simulink subsystem "RT_RelativeWindOnBlade"  (R2025a)
settings: Solver=VariableStepAuto  StartTime=0.0  StopTime=10.0  RelTol=1e-3
undefined symbols (not defined in the file): RT_BEDistFromEffSta_A, RT_BladeSegment_P, RT_HubOffsetBody_P, RT_ShaftTiltFwd_P, RT_ShaftTiltRight_P
settings Model: DataDictionary=Rotor.sldd  EnableAccessToBaseWorkspace=off  DefaultTestHarness=RT_RelativeWindOnBlade_Harness  Creator=tunglt60  LastModifiedBy=tunglt60

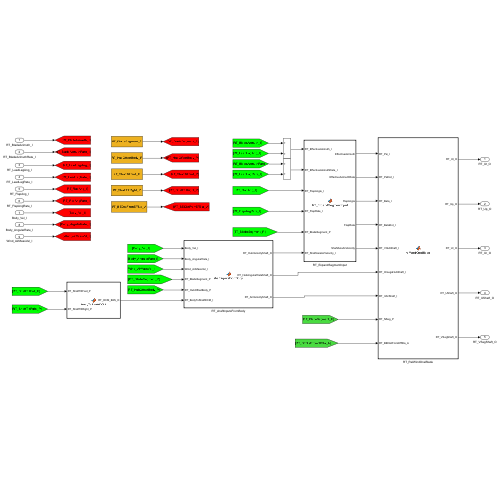
[thumbnail: Simulink's stored preview of the top-level diagram]
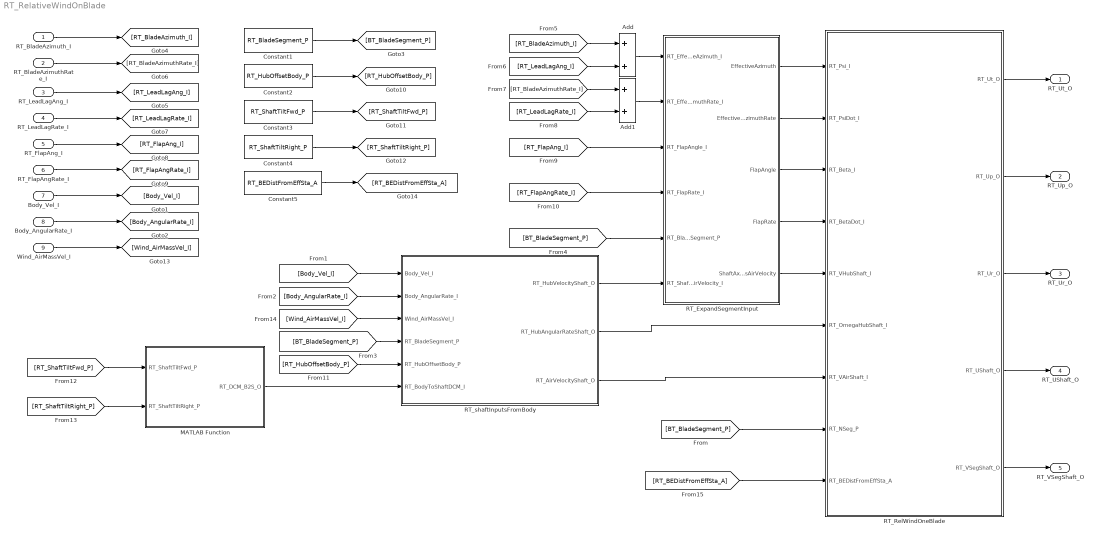
== system RT_RelativeWindOnBlade ==
  RT_BladeAzimuth_I : Inport
  RT_BladeAzimuthRate_I : Inport  Port=2
  RT_LeadLagAng_I : Inport  Port=3
  RT_LeadLagRate_I : Inport  Port=4
  RT_FlapAng_I : Inport  Port=5
  RT_FlapAngRate_I : Inport  Port=6
  Body_Vel_I : Inport  Port=7
  Body_AngularRate_I : Inport  Port=8
  Wind_AirMassVel_I : Inport  Port=9
  Add : Sum
  Add1 : Sum
  Constant1 : Constant  Value=RT_BladeSegment_P
  Constant2 : Constant  Value=RT_HubOffsetBody_P
  Constant3 : Constant  Value=RT_ShaftTiltFwd_P
  Constant4 : Constant  Value=RT_ShaftTiltRight_P
  Constant5 : Constant  Value=RT_BEDistFromEffSta_A
  MATLAB Function : MATLAB Function  TreatAsAtomicUnit=on
  RT_ExpandSegmentInput : MATLAB Function  TreatAsAtomicUnit=on
  RT_RelWindOneBlade : MATLAB Function  TreatAsAtomicUnit=on
  RT_shaftInputsFromBody : MATLAB Function  TreatAsAtomicUnit=on
  RT_Ut_O : Outport
  RT_Up_O : Outport  Port=2
  RT_Ur_O : Outport  Port=3
  RT_UShaft_O : Outport  Port=4
  RT_VSegShaft_O : Outport  Port=5
  wires:
  Add/1 -> RT_ExpandSegmentInput/1(RT_EffectiveAzimuth_I)
  Add1/1 -> RT_ExpandSegmentInput/2(RT_EffectiveAzimuthRate_I)
  Constant1/1 -> [BT_BladeSegment_P]
  [BT_BladeSegment_P] -> RT_ExpandSegmentInput/5(RT_BladeSegment_P)
  RT_BladeAzimuth_I/1 -> [RT_BladeAzimuth_I]
  RT_LeadLagRate_I/1 -> [RT_LeadLagRate_I]
  RT_FlapAngRate_I/1 -> [RT_FlapAngRate_I]
  RT_BladeAzimuthRate_I/1 -> [RT_BladeAzimuthRate_I]
  RT_LeadLagAng_I/1 -> [RT_LeadLagAng_I]
  RT_FlapAng_I/1 -> [RT_FlapAng_I]
  [RT_LeadLagAng_I] -> Add/2
  [RT_BladeAzimuth_I] -> Add/1
  [RT_BladeAzimuthRate_I] -> Add1/1
  [RT_LeadLagRate_I] -> Add1/2
  [RT_FlapAng_I] -> RT_ExpandSegmentInput/3(RT_FlapAngle_I)
  [RT_FlapAngRate_I] -> RT_ExpandSegmentInput/4(RT_FlapRate_I)
  Constant2/1 -> [RT_HubOffsetBody_P]
  Constant3/1 -> [RT_ShaftTiltFwd_P]
  Constant4/1 -> [RT_ShaftTiltRight_P]
  RT_ExpandSegmentInput/1(EffectiveAzimuth) -> RT_RelWindOneBlade/1(RT_Psi_I)
  RT_ExpandSegmentInput/2(EffectiveAzimuthRate) -> RT_RelWindOneBlade/2(RT_PsiDot_I)
  RT_ExpandSegmentInput/3(FlapAngle) -> RT_RelWindOneBlade/3(RT_Beta_I)
  RT_ExpandSegmentInput/4(FlapRate) -> RT_RelWindOneBlade/4(RT_BetaDot_I)
  [RT_ShaftTiltRight_P] -> MATLAB Function/2(RT_ShaftTiltRight_P)
  MATLAB Function/1(RT_DCM_B2S_O) -> RT_shaftInputsFromBody/6(RT_BodyToShaftDCM_I)
  [RT_ShaftTiltFwd_P] -> MATLAB Function/1(RT_ShaftTiltFwd_P)
  [BT_BladeSegment_P] -> RT_shaftInputsFromBody/4(RT_BladeSegment_P)
  [RT_HubOffsetBody_P] -> RT_shaftInputsFromBody/5(RT_HubOffsetBody_P)
  RT_shaftInputsFromBody/1(RT_HubVelocityShaft_O) -> RT_ExpandSegmentInput/6(RT_ShaftAxisAirVelocity_I)
  RT_shaftInputsFromBody/2(RT_HubAngularRateShaft_O) -> RT_RelWindOneBlade/6(RT_OmegaHubShaft_I)
  RT_shaftInputsFromBody/3(RT_AirVelocityShaft_O) -> RT_RelWindOneBlade/7(RT_VAirShaft_I)
  RT_ExpandSegmentInput/5(ShaftAxisAirVelocity) -> RT_RelWindOneBlade/5(RT_VHubShaft_I)
  [BT_BladeSegment_P] -> RT_RelWindOneBlade/8(RT_NSeg_P)
  Body_Vel_I/1 -> [Body_Vel_I]
  [Body_Vel_I] -> RT_shaftInputsFromBody/1(Body_Vel_I)
  Body_AngularRate_I/1 -> [Body_AngularRate_I]
  [Body_AngularRate_I] -> RT_shaftInputsFromBody/2(Body_AngularRate_I)
  [Wind_AirMassVel_I] -> RT_shaftInputsFromBody/3(Wind_AirMassVel_I)
  Wind_AirMassVel_I/1 -> [Wind_AirMassVel_I]
  [RT_BEDistFromEffSta_A] -> RT_RelWindOneBlade/9(RT_BEDistFromEffSta_A)
  Constant5/1 -> [RT_BEDistFromEffSta_A]
  RT_RelWindOneBlade/1(RT_Ut_O) -> RT_Ut_O/1
  RT_RelWindOneBlade/2(RT_Up_O) -> RT_Up_O/1
  RT_RelWindOneBlade/3(RT_Ur_O) -> RT_Ur_O/1
  RT_RelWindOneBlade/4(RT_UShaft_O) -> RT_UShaft_O/1
  RT_RelWindOneBlade/5(RT_VSegShaft_O) -> RT_VSegShaft_O/1

== matlab function RT_RelativeWindOnBlade/RT_shaftInputsFromBody ==
  data: Body_Vel_I input; RT_HubVelocityShaft_O output; Body_AngularRate_I input; Wind_AirMassVel_I input; RT_BladeSegment_P input; RT_HubAngularRateShaft_O output; RT_AirVelocityShaft_O output; RT_HubOffsetBody_P input; RT_BodyToShaftDCM_I input
function [RT_HubVelocityShaft_O, RT_HubAngularRateShaft_O, ...
    RT_AirVelocityShaft_O] = shaftInputsFromBody( ...
    Body_Vel_I, Body_AngularRate_I, ...
    Wind_AirMassVel_I, RT_BladeSegment_P, RT_HubOffsetBody_P, RT_BodyToShaftDCM_I)
%
% Convert body-axis quantities to shaft-axis quantities at rotor hub.
%
% Conventions:
%   body : x forward, y right, z down
%   shaft: z_s down along rotor shaft
%
% Inputs:
%   RT_ReferenceVelocityBody_I : [3x1], translational velocity of reference point
%                                in body axes (usually CG or body-origin)
%   RT_BodyAngularRate_I       : [3x1], body angular rate [p;q;r] in body axes
%   RT_AirMassVelocityBody_I   : [3x1] or [3xNSEG], air-mass velocity in body axes
%                                (NOT relative wind, NOT already minus vehicle velocity)
%   RT_BladeSegment_P
%   RT_HubOffsetBody_P      [3x1]
%   RT_BodyToShaftDCM_P     [3x3]
%
% Outputs:
%   RT_HubVelocityShaft_O      : [3x1], hub translational velocity in shaft axes
%   RT_HubAngularRateShaft_O   : [3x1], shaft angular rate in shaft axes
%   RT_AirVelocityShaft_O      : [3xNSEG], air-mass velocity in shaft axes
%
% Notes:
%   - If the reference point is already the hub, set:
%         RT_RotorParameter_I.RT_HubOffsetBody_P = [0;0;0]
%   - This assumes shaft is fixed to body.
%     If shaft rotates relative to body, add that relative rate separately.
%

NSEG = RT_BladeSegment_P;
C_SB   = RT_BodyToShaftDCM_I;
rHub_B = RT_HubOffsetBody_P;

% Hub translational velocity in body axes
Vhub_B = Body_Vel_I + cross(Body_AngularRate_I, rHub_B);

% Shaft fixed to body:
Whub_B = Body_AngularRate_I;

% Rotate to shaft axes
RT_HubVelocityShaft_O    = C_SB * Vhub_B;
RT_HubAngularRateShaft_O = C_SB * Whub_B;

% Air-mass velocity: expand to 3xNSEG if needed, then rotate each column
Vair_B = expand3xN(Wind_AirMassVel_I, NSEG);
RT_AirVelocityShaft_O = zeros(3, NSEG);

for k = 1:NSEG
    RT_AirVelocityShaft_O(:,k) = C_SB * Vair_B(:,k);
end

end

function Y = expand3xN(X, N)
%#codegen
if size(X,2) == 1
    Y = zeros(3, N);
    for i = 1:N
        Y(:,i) = X;
    end
else
    Y = X;
end
end

== matlab function RT_RelativeWindOnBlade/RT_RelWindOneBlade ==
  data: RT_Psi_I input; RT_Ut_O output; RT_PsiDot_I input; RT_Beta_I input; RT_BetaDot_I input; RT_VHubShaft_I input; RT_OmegaHubShaft_I input; RT_VAirShaft_I input; RT_NSeg_P input; RT_Up_O output; RT_Ur_O output; RT_UShaft_O output; RT_VSegShaft_O output; RT_BEDistFromEffSta_A input
function [RT_Ut_O, RT_Up_O, RT_Ur_O, RT_UShaft_O, RT_VSegShaft_O] = relWindOneBlade( ...
    RT_Psi_I, RT_PsiDot_I, RT_Beta_I, RT_BetaDot_I, ...
    RT_VHubShaft_I, RT_OmegaHubShaft_I, RT_VAirShaft_I, ...
    RT_NSeg_P, RT_BEDistFromEffSta_A)

    %
    % Compute relative wind at each blade element of one blade
    % (all vectors are expressed in shaft axes).
    %
    % Sign conventions:
    %   shaft +z points downward
    %   beta > 0 : flap up
    %   UT > 0   : opposite blade rotation direction
    %   UP > 0   : downward (shaft +z)
    %   UR > 0   : root -> tip
    %
    % Inputs:
    %   RT_Psi_I                : [1xNSEG], element azimuth angle [rad]
    %   RT_PsiDot_I             : [1xNSEG], azimuth rate [rad/s]
    %   RT_Beta_I               : [1xNSEG], flap angle [rad]
    %   RT_BetaDot_I            : [1xNSEG], flap rate [rad/s]
    %   RT_VHubShaft_I          : [3x1], hub translational velocity [m/s]
    %   RT_OmegaHubShaft_I      : [3x1], hub angular rate [rad/s]
    %   RT_VAirShaft_I          : [3xNSEG], local air velocity at element stations [m/s]
    %   RT_NSeg_P               : scalar, number of blade elements
    %   RT_BEDistFromEffSta_A   : [1xNSEG] or [NSEGx1], radius of each element station [m]
    %
    % Outputs:
    %   RT_Ut_O                 : [1xNSEG], tangential relative wind component UT [m/s]
    %   RT_Up_O                 : [1xNSEG], perpendicular relative wind component UP [m/s]
    %   RT_Ur_O                 : [1xNSEG], radial relative wind component UR [m/s]
    %   RT_UShaft_O             : [3xNSEG], relative wind vector in shaft axes [m/s]
    %   RT_VSegShaft_O          : [3xNSEG], absolute element velocity in shaft axes [m/s]
    
    nSeg = RT_NSeg_P;
    
    RT_Ut_O        = zeros(1, nSeg);
    RT_Up_O        = zeros(1, nSeg);
    RT_Ur_O        = zeros(1, nSeg);
    
    RT_UShaft_O    = zeros(3, nSeg);
    RT_VSegShaft_O = zeros(3, nSeg);
    
    ez = [0; 0; 1];   % +z_shaft is DOWN
    
    for k = 1:nSeg
        rk = RT_BEDistFromEffSta_A(k);
    
        psi   = RT_Psi_I(k);
        dpsi  = RT_PsiDot_I(k);
        beta  = RT_Beta_I(k);
        dbeta = RT_BetaDot_I(k);
    
        cp = cos(psi);
        sp = sin(psi);
        cb = cos(beta);
        sb = sin(beta);
    
        eR0 = [cp; sp; 0.0];
        eA  = [-sp; cp; 0.0];
    
        eR = cb * eR0 - sb * ez;
        eP = cross(eR, eA);
        eT = -signNoZero(dpsi) * eA;
    
        rSeg = rk * eR;
        vRel = rk * cb * dpsi * eA - rk * dbeta * eP;
    
        RT_VSegShaft_O(:, k) = RT_VHubShaft_I + ...
            cross(RT_OmegaHubShaft_I, rSeg) + vRel;
    
        u = RT_VAirShaft_I(:, k) - RT_VSegShaft_O(:, k);
        RT_UShaft_O(:, k) = u;
    
        RT_Ut_O(k) = dot(u, eT);  % UT > 0 opposite rotation
        RT_Up_O(k) = dot(u, eP);  % UP > 0 down
        RT_Ur_O(k) = dot(u, eR);  % UR > 0 root -> tip
    end
end

== matlab function RT_RelativeWindOnBlade/RT_ExpandSegmentInput ==
  data: RT_EffectiveAzimuth_I input; EffectiveAzimuth output; RT_EffectiveAzimuthRate_I input; RT_FlapAngle_I input; RT_FlapRate_I input; RT_BladeSegment_P input; EffectiveAzimuthRate output; FlapAngle output; FlapRate output; ShaftAxisAirVelocity output; RT_ShaftAxisAirVelocity_I input
function [EffectiveAzimuth, EffectiveAzimuthRate, ...
    FlapAngle, FlapRate, ShaftAxisAirVelocity] = RT_ExpandSegmentInput(RT_EffectiveAzimuth_I, ...
    RT_EffectiveAzimuthRate_I, RT_FlapAngle_I, RT_FlapRate_I, RT_BladeSegment_P, RT_ShaftAxisAirVelocity_I)

NSEG = RT_BladeSegment_P;

% Expand scalars to 1xNSEG
EffectiveAzimuth     = expand1xN(RT_EffectiveAzimuth_I, NSEG);
EffectiveAzimuthRate = expand1xN(RT_EffectiveAzimuthRate_I, NSEG);
FlapAngle            = expand1xN(RT_FlapAngle_I, NSEG);
FlapRate             = expand1xN(RT_FlapRate_I, NSEG);

% Expand Vair if needed
ShaftAxisAirVelocity = expand3xN(RT_ShaftAxisAirVelocity_I, NSEG);


end

function y = expand1xN(x, n)
%#codegen
if isscalar(x)
    y = zeros(1, n);
    for i = 1:n
        y(i) = x;
    end
else
    y = reshape(x, 1, n);
end
end

function Y = expand3xN(X, n)
%#codegen
if size(X, 2) == 1
    Y = zeros(3, n);
    for i = 1:n
        Y(:,i) = X;
    end
else
    Y = X;
end
end

== matlab function RT_RelativeWindOnBlade/MATLAB Function ==
  data: RT_ShaftTiltFwd_P input; RT_DCM_B2S_O output; RT_ShaftTiltRight_P input
function RT_DCM_B2S_O  = bodyToShaftDCM( ...
    RT_ShaftTiltFwd_P, RT_ShaftTiltRight_P)
%
% Build DCM body -> shaft from shaft tilt.
%
% Positive angles mean:
%   RT_ShaftTiltFwd_I   > 0 : top of shaft tilts forward
%   RT_ShaftTiltRight_I > 0 : top of shaft tilts right
%
% If your convention is instead "+z_s tilts forward/right",
% negate the two inputs.
%

cF = cos(RT_ShaftTiltFwd_P);
sF = sin(RT_ShaftTiltFwd_P);
cR = cos(RT_ShaftTiltRight_P);
sR = sin(RT_ShaftTiltRight_P);

% Shaft basis expressed in body axes
DCM_S2B = [  cF,       0.0,   -sF;
             -sR*sF,   cR,    -sR*cF;
              cR*sF,   sR,     cR*cF ];

RT_DCM_B2S_O = DCM_S2B.';
end
